simulink model "PIDSimulinkDrawing"  (R2016a)
settings: Solver=VariableStepAuto  StartTime=0.0  StopTime=10.0  RelTol=1e-3
undefined symbols (not defined in the file): KD, KI, KP, Recv
settings Model: Creator=Lenovo  LastModifiedBy=Lenovo

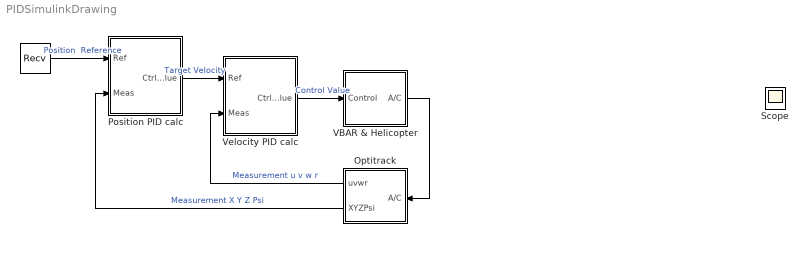
== system PIDSimulinkDrawing ==
  " " : Constant  Value=Recv
  Optitrack : Subsystem
  Position PID calc : Subsystem
  Scope : Scope
  VBAR & Helicopter : Subsystem
  Velocity PID calc : Subsystem
  wires:
  " "/1 -> Position PID calc/1(Ref)  "Position  Reference"
  Optitrack/2(XYZPsi) -> Position PID calc/2(Meas)  "Measurement X Y Z Psi"
  Position PID calc/1(Ctrl_Value) -> Velocity PID calc/1(Ref)  "Target Velocity"
  Optitrack/1(uvwr) -> Velocity PID calc/2(Meas)  "Measurement u v w r"
  Velocity PID calc/1(Ctrl_Value) -> VBAR & Helicopter/1(Control)  "Control Value"
  VBAR & Helicopter/1(A/C) -> Optitrack/1(A/C)

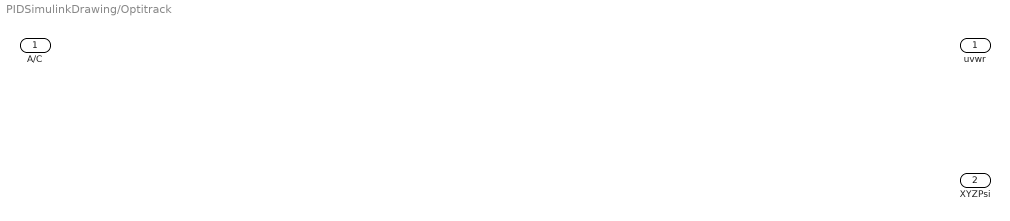
== system PIDSimulinkDrawing/Optitrack ==
  A/C : Inport
  uvwr : Outport
  XYZPsi : Outport  Port=2

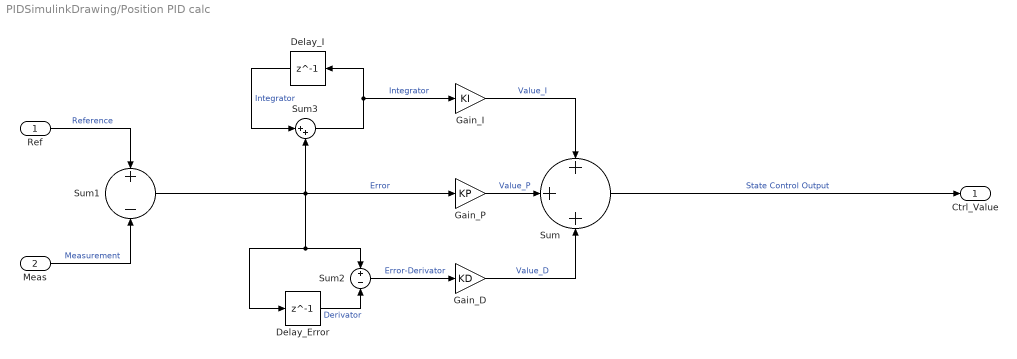
== system PIDSimulinkDrawing/Position PID calc ==
  Ref : Inport
  Meas : Inport  Port=2
  Delay_Error : Delay  DelayLength=1
  Delay_I : Delay  DelayLength=1
  Gain_D : Gain  Gain=KD
  Gain_I : Gain  Gain=KI
  Gain_P : Gain  Gain=KP
  Sum : Sum  Inputs=+++
  Sum1 : Sum  Inputs=+|-
  Sum2 : Sum  Inputs=+|-
  Sum3 : Sum  Inputs=|++
  Ctrl_Value : Outport
  wires:
  Gain_P/1 -> Sum/2  "Value_P"
  Gain_D/1 -> Sum/3  "Value_D"
  Sum2/1 -> Gain_D/1  "Error-Derivator"
  Delay_Error/1 -> Sum2/2  "Derivator"
  Delay_I/1 -> Sum3/1  "Integrator"
  Gain_I/1 -> Sum/1  "Value_I"
  Sum/1 -> Ctrl_Value/1  "State Control Output"
  Sum3/1 -> Delay_I/1, Gain_I/1  "Integrator"
  Ref/1 -> Sum1/1  "Reference"
  Meas/1 -> Sum1/2  "Measurement"
  Sum1/1 -> Delay_Error/1, Sum2/1, Gain_P/1, Sum3/2  "Error"

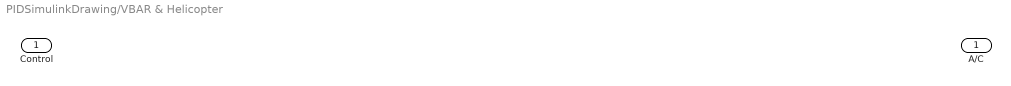
== system PIDSimulinkDrawing/VBAR & Helicopter ==
  Control : Inport
  A/C : Outport

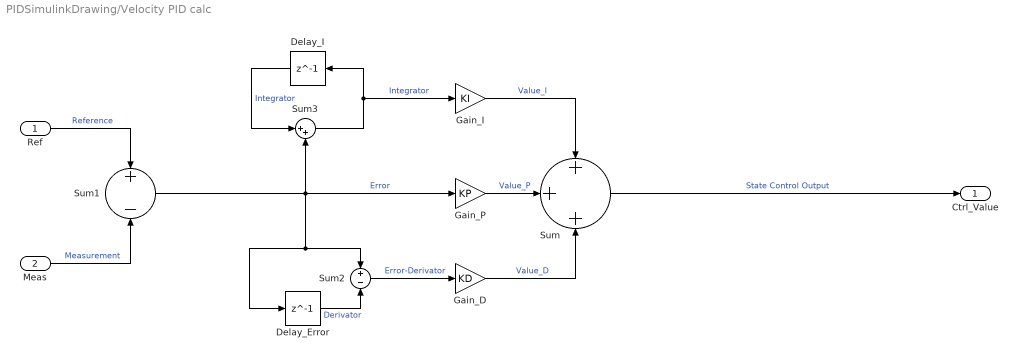
== system PIDSimulinkDrawing/Velocity PID calc ==
  Ref : Inport
  Meas : Inport  Port=2
  Delay_Error : Delay  DelayLength=1
  Delay_I : Delay  DelayLength=1
  Gain_D : Gain  Gain=KD
  Gain_I : Gain  Gain=KI
  Gain_P : Gain  Gain=KP
  Sum : Sum  Inputs=+++
  Sum1 : Sum  Inputs=+|-
  Sum2 : Sum  Inputs=+|-
  Sum3 : Sum  Inputs=|++
  Ctrl_Value : Outport
  wires:
  Gain_P/1 -> Sum/2  "Value_P"
  Gain_D/1 -> Sum/3  "Value_D"
  Sum2/1 -> Gain_D/1  "Error-Derivator"
  Delay_Error/1 -> Sum2/2  "Derivator"
  Delay_I/1 -> Sum3/1  "Integrator"
  Gain_I/1 -> Sum/1  "Value_I"
  Sum/1 -> Ctrl_Value/1  "State Control Output"
  Sum3/1 -> Delay_I/1, Gain_I/1  "Integrator"
  Ref/1 -> Sum1/1  "Reference"
  Meas/1 -> Sum1/2  "Measurement"
  Sum1/1 -> Delay_Error/1, Sum2/1, Gain_P/1, Sum3/2  "Error"
